simulink model "simulator_PID"  (R2024b)
settings: Solver=FixedStepAuto  StartTime=0.0  StopTime=100  FixedStep=0.01  RelTol=1e-3
values from neighbouring files (symbols this model uses):
  g = system_params.g    [system_model_quarternions.m]    (also in system_model_quat_omega.m)
  m = size(B,2)    [discretize_system.m]    (also in linearize_system.m = length(u0); linearize_system_euler.m = length(u0); model_init.m = system_params.m; system_model_quarternions.m = system_params.m)
  q0 = [0; 0; 0]    [model_init.m]    (also in test_model.m = x_test(1:3))
  qdot0 = [0;0;0]    [model_init.m]
  W_inv = inv(system_params.W)    [model_init.m]
undefined symbols (not defined in the file or in its folder): ALR, AUR, FD, LD, Lh, PLR, PUR, RD, W
libraries: slpidlib x5
settings Model: Creator=Sigbjørn  LastModifiedBy=Sigbjørn

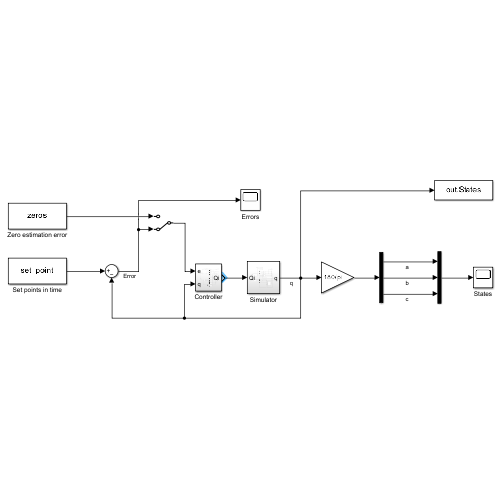
[thumbnail: Simulink's stored preview of the top-level diagram]
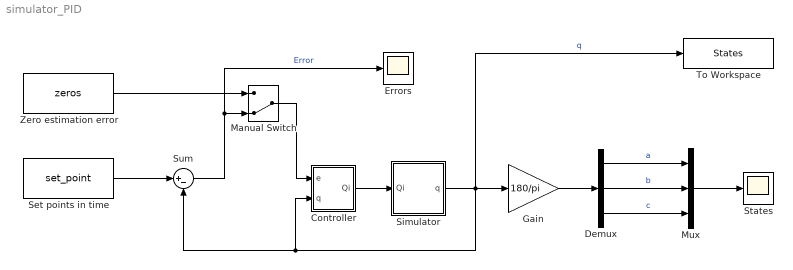
== system simulator_PID ==
  Controller : Subsystem
  Demux : Demux  Outputs=3
  Errors : Scope
  Gain : Gain  Gain=180/pi
  Manual Switch : ManualSwitch  CurrentSetting=0
  Mux : Mux  Inputs=3
  Set points in time : FromWorkspace  VariableName=set_point
  Simulator : Subsystem
  States : Scope
  Sum : Sum  Inputs=|+-
  To Workspace : ToWorkspace  VariableName=States  SaveFormat=Timeseries  SampleTime=-1
  Zero estimation error : FromWorkspace  VariableName=zeros
  wires:
  Set points in time/1 -> Sum/1
  Controller/1(Qi) -> Simulator/1(Qi)
  Sum/1 -> Manual Switch/2, Errors/1  "Error"
  Simulator/1(q) -> To Workspace/1, Gain/1, Controller/2(q), Sum/2  "q"
  Demux/1 -> Mux/1  "a"
  Demux/2 -> Mux/2  "b"
  Demux/3 -> Mux/3  "c"
  Zero estimation error/1 -> Manual Switch/1
  Manual Switch/1 -> Controller/1(e)
  Gain/1 -> Demux/1
  Mux/1 -> States/1

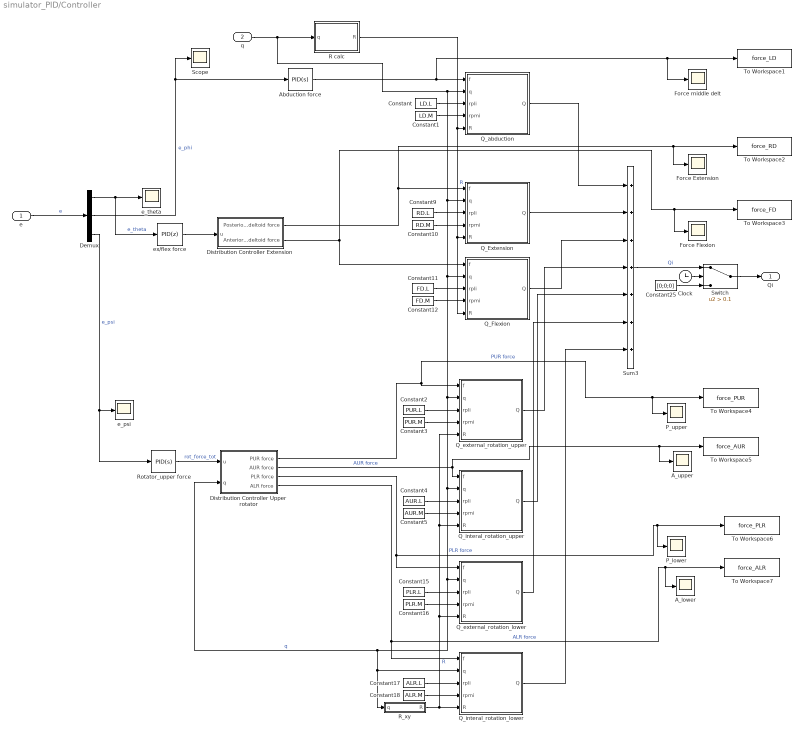
== system simulator_PID/Controller ==
  e : Inport
  q : Inport  Port=2
  A_lower : Scope
  A_upper : Scope
  Abduction force : slpidlib/PID Controller  Controller=PID  Form=Parallel  TimeDomain=Continuous-time  UseExternalTs=off  SampleTime=-1  IntegratorMethod=Forward Euler  FilterMethod=Forward Euler  ControllerParametersSource=internal  P=1  I=25  UseKiTs=off  D=5  UseExternalDerivativeSource=off  N=100  UseFilter=on  TunerSelectOption=Transfer Function Based (PID Tuner App)  InitialConditionSource=internal  InitialConditionForIntegrator=0  InitialConditionForFilter=0  DifferentiatorICPrevScaledInput=0  ExternalReset=none  TrackingMode=off  Kt=1  LimitOutput=on  SatLimitsSource=internal  UpperSaturationLimit=inf  LowerSaturationLimit=0  LinearizeAsGain=on  AntiWindupMode=none  Kb=1  LimitIntegrator=on  UpperIntegratorSaturationLimit=10000  LowerIntegratorSaturationLimit=0  POutMin=[]  POutMax=[]  IOutMin=[]  IOutMax=[]  DOutMin=[]  DOutMax=[]  NOutMin=[]  NOutMax=[]  SumOutMin=[]  SumOutMax=[]  SaturationOutMin=[]  SaturationOutMax=[]  PParamMin=[]  PParamMax=[]  IParamMin=[]  IParamMax=[]  DParamMin=[]  DParamMax=[]  NParamMin=[]  NParamMax=[]  KbParamMin=[]  KbParamMax=[]  KtParamMin=[]  KtParamMax=[]  KbOutMin=[]  KbOutMax=[]  KtOutMin=[]  KtOutMax=[]  IntegratorOutMin=[]  IntegratorOutMax=[]  FilterOutMin=[]  FilterOutMax=[]  SumI1OutMin=[]  SumI1OutMax=[]  SumI2OutMin=[]  SumI2OutMax=[]  SumI3OutMin=[]  SumI3OutMax=[]  SumI4OutMin=[]  SumI4OutMax=[]  SumDOutMin=[]  SumDOutMax=[]  DifferentiatorOutMin=[]  DifferentiatorOutMax=[]  FilterDiffOutCoefMin=[]  FilterDiffOutCoefMax=[]  ReciprocalOutMin=[]  ReciprocalOutMax=[]  SumDenOutMin=[]  SumDenOutMax=[]  SumNumOutMin=[]  SumNumOutMax=[]  DivideOutMin=[]  DivideOutMax=[]  UdiffTsProdOutMin=[]  UdiffTsProdOutMax=[]  NTsProdOutMin=[]  NTsProdOutMax=[]  UintegralTsProdOutMin=[]  UintegralTsProdOutMax=[]  UngainTsProdOutMin=[]  UngainTsProdOutMax=[]  ClampingZeroOutDataTypeStr=Inherit: Inherit via back propagation  ClampingZeroOutMin=[]  ClampingZeroOutMax=[]  FilterDenConstantOutDataTypeStr=Inherit: Inherit via back propagation  FilterDenConstantOutMin=[]  FilterDenConstantOutMax=[]  PCopyOutDataTypeStr=Inherit: Inherit via back propagation  PCopyOutMin=[]  PCopyOutMax=[]  NCopyOutDataTypeStr=Inherit: Inherit via back propagation  NCopyOutMin=[]  NCopyOutMax=[]  IntegratorContinuousStateAttributes=''  IntegratorStateMustResolveToSignalObject=off  IntegratorRTWStateStorageClass=Auto  FilterContinuousStateAttributes=''  FilterStateMustResolveToSignalObject=off  FilterRTWStateStorageClass=Auto  ParallelPVariant=InternalParameters  IdealPVariant=Disabled  IVariant=InternalParameters  DVariant=InternalParameters  IntegratorVariant=Continuous  SatVariant=Enabled  AWVariant=Passthrough  PCopyVariant=Disabled  TRVariant=Disabled  FdbkBlocksVariant=Forward  IdealPFdbkVariant=Disabled  SatFdbkVariant=Disabled  DerivativeFilterVariant=ContFilter  NVariant=InternalParameters  NCopyVariant=Disabled  FilterICVariant=InternalICsFilter  IntegratorICVariant=InternalICs  ExternalResetVariant=Disabled  TRSumVariant=Passthrough  SumFdbkVariant=Disabled  SumVariant=Sum_PID  TsampFilterVariant=InternalTs  TsampNgainVariant=Passthrough  TsampIntegralVariant=Disabled_SignalSpec  ExternalSaturationOutDataTypeStr=Inherit: Same as second input  DerivativeSourceVariant=ErrorSignal  PreIntVariant=InternalPreInt
  Clock : Clock
  Constant : Constant  Value=LD.L
  Constant1 : Constant  Value=LD.M
  Constant10 : Constant  Value=RD.M
  Constant11 : Constant  Value=FD.L
  Constant12 : Constant  Value=FD.M
  Constant15 : Constant  Value=PLR.L
  Constant16 : Constant  Value=PLR.M
  Constant17 : Constant  Value=ALR.L
  Constant18 : Constant  Value=ALR.M
  Constant2 : Constant  Value=PUR.L
  Constant25 : Constant  Value=[0;0;0]
  Constant3 : Constant  Value=PUR.M
  Constant4 : Constant  Value=AUR.L
  Constant5 : Constant  Value=AUR.M
  Constant9 : Constant  Value=RD.L
  Demux : Demux  Outputs=3
  Distribution Controller Extension : Subsystem
  Distribution Controller Upper rotator : Subsystem
  Force Extension : Scope
  Force Flexion : Scope
  Force middle delt : Scope
  P_lower : Scope
  P_upper : Scope
  Q_Extension : MATLAB Function  TreatAsAtomicUnit=on
  Q_Flexion : MATLAB Function  TreatAsAtomicUnit=on
  Q_abduction : MATLAB Function  TreatAsAtomicUnit=on
  Q_external_rotation_lower : MATLAB Function  TreatAsAtomicUnit=on
  Q_external_rotation_upper : MATLAB Function  TreatAsAtomicUnit=on
  Q_interal_rotation_lower : MATLAB Function  TreatAsAtomicUnit=on
  Q_interal_rotation_upper : MATLAB Function  TreatAsAtomicUnit=on
  R calc : MATLAB Function  TreatAsAtomicUnit=on
  R_xy : MATLAB Function  TreatAsAtomicUnit=on
  Rotator_upper force : slpidlib/PID Controller  Controller=PID  Form=Parallel  TimeDomain=Continuous-time  UseExternalTs=off  SampleTime=-1  IntegratorMethod=Forward Euler  FilterMethod=Forward Euler  ControllerParametersSource=internal  P=100  I=200  UseKiTs=off  D=500  UseExternalDerivativeSource=off  N=100  UseFilter=on  TunerSelectOption=Transfer Function Based (PID Tuner App)  InitialConditionSource=internal  InitialConditionForIntegrator=0  InitialConditionForFilter=0  DifferentiatorICPrevScaledInput=0  ExternalReset=none  TrackingMode=off  Kt=1  LimitOutput=on  SatLimitsSource=internal  UpperSaturationLimit=inf  LowerSaturationLimit=-inf  LinearizeAsGain=on  AntiWindupMode=none  Kb=1  LimitIntegrator=on  UpperIntegratorSaturationLimit=inf  LowerIntegratorSaturationLimit=-inf  POutMin=[]  POutMax=[]  IOutMin=[]  IOutMax=[]  DOutMin=[]  DOutMax=[]  NOutMin=[]  NOutMax=[]  SumOutMin=[]  SumOutMax=[]  SaturationOutMin=[]  SaturationOutMax=[]  PParamMin=[]  PParamMax=[]  IParamMin=[]  IParamMax=[]  DParamMin=[]  DParamMax=[]  NParamMin=[]  NParamMax=[]  KbParamMin=[]  KbParamMax=[]  KtParamMin=[]  KtParamMax=[]  KbOutMin=[]  KbOutMax=[]  KtOutMin=[]  KtOutMax=[]  IntegratorOutMin=[]  IntegratorOutMax=[]  FilterOutMin=[]  FilterOutMax=[]  SumI1OutMin=[]  SumI1OutMax=[]  SumI2OutMin=[]  SumI2OutMax=[]  SumI3OutMin=[]  SumI3OutMax=[]  SumI4OutMin=[]  SumI4OutMax=[]  SumDOutMin=[]  SumDOutMax=[]  DifferentiatorOutMin=[]  DifferentiatorOutMax=[]  FilterDiffOutCoefMin=[]  FilterDiffOutCoefMax=[]  ReciprocalOutMin=[]  ReciprocalOutMax=[]  SumDenOutMin=[]  SumDenOutMax=[]  SumNumOutMin=[]  SumNumOutMax=[]  DivideOutMin=[]  DivideOutMax=[]  UdiffTsProdOutMin=[]  UdiffTsProdOutMax=[]  NTsProdOutMin=[]  NTsProdOutMax=[]  UintegralTsProdOutMin=[]  UintegralTsProdOutMax=[]  UngainTsProdOutMin=[]  UngainTsProdOutMax=[]  ClampingZeroOutDataTypeStr=Inherit: Inherit via back propagation  ClampingZeroOutMin=[]  ClampingZeroOutMax=[]  FilterDenConstantOutDataTypeStr=Inherit: Inherit via back propagation  FilterDenConstantOutMin=[]  FilterDenConstantOutMax=[]  PCopyOutDataTypeStr=Inherit: Inherit via back propagation  PCopyOutMin=[]  PCopyOutMax=[]  NCopyOutDataTypeStr=Inherit: Inherit via back propagation  NCopyOutMin=[]  NCopyOutMax=[]  IntegratorContinuousStateAttributes=''  IntegratorStateMustResolveToSignalObject=off  IntegratorRTWStateStorageClass=Auto  FilterContinuousStateAttributes=''  FilterStateMustResolveToSignalObject=off  FilterRTWStateStorageClass=Auto  ParallelPVariant=InternalParameters  IdealPVariant=Disabled  IVariant=InternalParameters  DVariant=InternalParameters  IntegratorVariant=Continuous  SatVariant=Enabled  AWVariant=Passthrough  PCopyVariant=Disabled  TRVariant=Disabled  FdbkBlocksVariant=Forward  IdealPFdbkVariant=Disabled  SatFdbkVariant=Disabled  DerivativeFilterVariant=ContFilter  NVariant=InternalParameters  NCopyVariant=Disabled  FilterICVariant=InternalICsFilter  IntegratorICVariant=InternalICs  ExternalResetVariant=Disabled  TRSumVariant=Passthrough  SumFdbkVariant=Disabled  SumVariant=Sum_PID  TsampFilterVariant=InternalTs  TsampNgainVariant=Passthrough  TsampIntegralVariant=Disabled_SignalSpec  ExternalSaturationOutDataTypeStr=Inherit: Same as second input  DerivativeSourceVariant=ErrorSignal  PreIntVariant=InternalPreInt
  Scope : Scope
  Sum3 : Sum  Inputs=+++++++  InputSameDT=on  SaturateOnIntegerOverflow=on  OutDataTypeStr=Inherit: Same as first input
  Switch : Switch  Criteria=u2 > Threshold  Threshold=0.1  SaturateOnIntegerOverflow=off  InputSameDT=off
  To Workspace1 : ToWorkspace  VariableName=force_LD  SaveFormat=Timeseries  SampleTime=-1
  To Workspace2 : ToWorkspace  VariableName=force_RD  SaveFormat=Timeseries  SampleTime=-1
  To Workspace3 : ToWorkspace  VariableName=force_FD  SaveFormat=Timeseries  SampleTime=-1
  To Workspace4 : ToWorkspace  VariableName=force_PUR  SaveFormat=Timeseries  SampleTime=-1
  To Workspace5 : ToWorkspace  VariableName=force_AUR  SaveFormat=Timeseries  SampleTime=-1
  To Workspace6 : ToWorkspace  VariableName=force_PLR  SaveFormat=Timeseries  SampleTime=-1
  To Workspace7 : ToWorkspace  VariableName=force_ALR  SaveFormat=Timeseries  SampleTime=-1
  e_psi : Scope
  e_theta : Scope
  ex/flex force : slpidlib/PID Controller  Controller=PID  Form=Parallel  TimeDomain=Discrete-time  UseExternalTs=off  SampleTime=-1  IntegratorMethod=Forward Euler  FilterMethod=Forward Euler  ControllerParametersSource=internal  P=1  I=25  UseKiTs=off  D=5  UseExternalDerivativeSource=off  N=100  UseFilter=on  TunerSelectOption=Transfer Function Based (PID Tuner App)  InitialConditionSource=internal  InitialConditionForIntegrator=0  InitialConditionForFilter=0  DifferentiatorICPrevScaledInput=0  ExternalReset=none  TrackingMode=off  Kt=1  LimitOutput=on  SatLimitsSource=internal  UpperSaturationLimit=inf  LowerSaturationLimit=-inf  LinearizeAsGain=on  AntiWindupMode=none  Kb=1  LimitIntegrator=on  UpperIntegratorSaturationLimit=inf  LowerIntegratorSaturationLimit=-inf  POutMin=[]  POutMax=[]  IOutMin=[]  IOutMax=[]  DOutMin=[]  DOutMax=[]  NOutMin=[]  NOutMax=[]  SumOutMin=[]  SumOutMax=[]  SaturationOutMin=[]  SaturationOutMax=[]  PParamMin=[]  PParamMax=[]  IParamMin=[]  IParamMax=[]  DParamMin=[]  DParamMax=[]  NParamMin=[]  NParamMax=[]  KbParamMin=[]  KbParamMax=[]  KtParamMin=[]  KtParamMax=[]  KbOutMin=[]  KbOutMax=[]  KtOutMin=[]  KtOutMax=[]  IntegratorOutMin=[]  IntegratorOutMax=[]  FilterOutMin=[]  FilterOutMax=[]  SumI1OutMin=[]  SumI1OutMax=[]  SumI2OutMin=[]  SumI2OutMax=[]  SumI3OutMin=[]  SumI3OutMax=[]  SumI4OutMin=[]  SumI4OutMax=[]  SumDOutMin=[]  SumDOutMax=[]  DifferentiatorOutMin=[]  DifferentiatorOutMax=[]  FilterDiffOutCoefMin=[]  FilterDiffOutCoefMax=[]  ReciprocalOutMin=[]  ReciprocalOutMax=[]  SumDenOutMin=[]  SumDenOutMax=[]  SumNumOutMin=[]  SumNumOutMax=[]  DivideOutMin=[]  DivideOutMax=[]  UdiffTsProdOutMin=[]  UdiffTsProdOutMax=[]  NTsProdOutMin=[]  NTsProdOutMax=[]  UintegralTsProdOutMin=[]  UintegralTsProdOutMax=[]  UngainTsProdOutMin=[]  UngainTsProdOutMax=[]  ClampingZeroOutDataTypeStr=Inherit: Inherit via back propagation  ClampingZeroOutMin=[]  ClampingZeroOutMax=[]  FilterDenConstantOutDataTypeStr=Inherit: Inherit via back propagation  FilterDenConstantOutMin=[]  FilterDenConstantOutMax=[]  PCopyOutDataTypeStr=Inherit: Inherit via back propagation  PCopyOutMin=[]  PCopyOutMax=[]  NCopyOutDataTypeStr=Inherit: Inherit via back propagation  NCopyOutMin=[]  NCopyOutMax=[]  IntegratorContinuousStateAttributes=''  IntegratorStateMustResolveToSignalObject=off  IntegratorRTWStateStorageClass=Auto  FilterContinuousStateAttributes=''  FilterStateMustResolveToSignalObject=off  FilterRTWStateStorageClass=Auto  ParallelPVariant=InternalParameters  IdealPVariant=Disabled  IVariant=InternalParameters  DVariant=InternalParameters  IntegratorVariant=Discrete  SatVariant=Enabled  AWVariant=Passthrough  PCopyVariant=Disabled  TRVariant=Disabled  FdbkBlocksVariant=Forward  IdealPFdbkVariant=Disabled  SatFdbkVariant=Disabled  DerivativeFilterVariant=ForwardEulerFilter  NVariant=InternalParameters  NCopyVariant=Disabled  FilterICVariant=InternalICsFilter  IntegratorICVariant=InternalICs  ExternalResetVariant=Disabled  TRSumVariant=Passthrough  SumFdbkVariant=Disabled  SumVariant=Sum_PID  TsampFilterVariant=InternalTs  TsampNgainVariant=Passthrough  TsampIntegralVariant=Disabled_SignalSpec  ExternalSaturationOutDataTypeStr=Inherit: Same as second input  DerivativeSourceVariant=ErrorSignal  PreIntVariant=InternalPreInt
  Qi : Outport
  wires:
  q/1 -> Q_abduction/2(q), Q_Extension/2(q), Q_Flexion/2(q), Q_interal_rotation_lower/2(q), R_xy/1(q), Distribution Controller Upper rotator/2(q), Q_external_rotation_lower/2(q), Q_interal_rotation_upper/2(q), Q_external_rotation_upper/2(q), R calc/1(q)  "q"
  R calc/1(R) -> Q_Extension/5(R), Q_Flexion/5(R), Q_abduction/5(R)  "R"
  Constant/1 -> Q_abduction/3(rpli)
  Constant1/1 -> Q_abduction/4(rpmi)
  Sum3/1 -> Switch/1  "Qi"
  Demux/1 -> ex/flex force/1, e_theta/1  "e_theta"
  Demux/2 -> Scope/1, Abduction force/1  "e_phi"
  Demux/3 -> Rotator_upper force/1, e_psi/1  "e_psi"
  Constant2/1 -> Q_external_rotation_upper/3(rpli)
  Constant3/1 -> Q_external_rotation_upper/4(rpmi)
  Constant4/1 -> Q_interal_rotation_upper/3(rpli)
  Constant5/1 -> Q_interal_rotation_upper/4(rpmi)
  Q_abduction/1(Q) -> Sum3/1
  Q_interal_rotation_upper/1(Q) -> Sum3/5
  Q_external_rotation_upper/1(Q) -> Sum3/4
  Rotator_upper force/1 -> Distribution Controller Upper rotator/1(u)  "rot_force_tot"
  ex/flex force/1 -> Distribution Controller Extension/1(u)
  Constant9/1 -> Q_Extension/3(rpli)
  Constant10/1 -> Q_Extension/4(rpmi)
  Constant11/1 -> Q_Flexion/3(rpli)
  Constant12/1 -> Q_Flexion/4(rpmi)
  Q_Flexion/1(Q) -> Sum3/3
  Q_Extension/1(Q) -> Sum3/2
  Abduction force/1 -> Force middle delt/1, To Workspace1/1, Q_abduction/1(f)
  Distribution Controller Extension/1(Posterior deltoid force) -> To Workspace2/1, Force Extension/1, Q_Extension/1(f)
  Distribution Controller Extension/2(Anterior deltoid force) -> Q_Flexion/1(f), To Workspace3/1, Force Flexion/1
  Q_external_rotation_lower/1(Q) -> Sum3/6
  Q_interal_rotation_lower/1(Q) -> Sum3/7
  Constant15/1 -> Q_external_rotation_lower/3(rpli)
  Constant16/1 -> Q_external_rotation_lower/4(rpmi)
  Constant17/1 -> Q_interal_rotation_lower/3(rpli)
  Constant18/1 -> Q_interal_rotation_lower/4(rpmi)
  e/1 -> Demux/1  "e"
  Clock/1 -> Switch/2
  Constant25/1 -> Switch/3
  Switch/1 -> Qi/1
  Distribution Controller Upper rotator/4(ALR force) -> To Workspace7/1, A_lower/1, Q_interal_rotation_lower/1(f)  "ALR force"
  Distribution Controller Upper rotator/3(PLR force) -> To Workspace6/1, P_lower/1, Q_external_rotation_lower/1(f)  "PLR force"
  Distribution Controller Upper rotator/2(AUR force) -> A_upper/1, To Workspace5/1, Q_interal_rotation_upper/1(f)  "AUR force"
  Distribution Controller Upper rotator/1(PUR force) -> To Workspace4/1, P_upper/1, Q_external_rotation_upper/1(f)  "PUR force"
  R_xy/1(R) -> Q_external_rotation_upper/5(R), Q_interal_rotation_upper/5(R), Q_external_rotation_lower/5(R), Q_interal_rotation_lower/5(R)  "R"

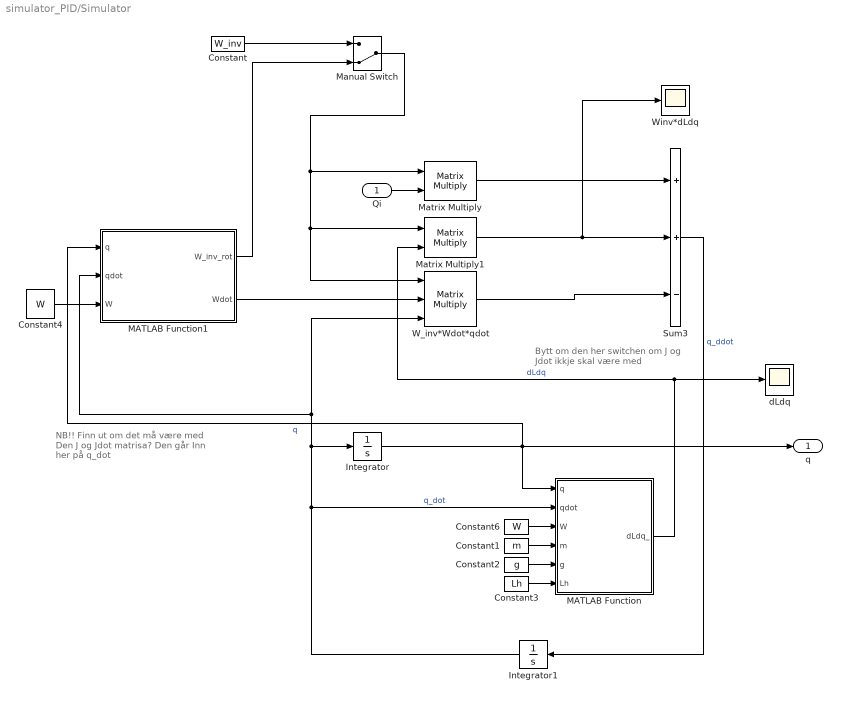
== system simulator_PID/Simulator ==
  note: Bytt om den her switchen
      | om J og Jdot ikkje skal være med
  note: NB!! Finn ut om det må være med
      | Den J og Jdot matrisa? Den går
      | Inn her på q_dot
  Qi : Inport
  Constant : Constant  Value=W_inv
  Constant1 : Constant  Value=m
  Constant2 : Constant  Value=g
  Constant3 : Constant  Value=Lh
  Constant4 : Constant  Value=W
  Constant6 : Constant  Value=W
  Integrator : Integrator  InitialCondition=q0
  Integrator1 : Integrator  InitialCondition=qdot0
  MATLAB Function : MATLAB Function  TreatAsAtomicUnit=on
  MATLAB Function1 : MATLAB Function  TreatAsAtomicUnit=on
  Manual Switch : ManualSwitch  CurrentSetting=0
  Matrix Multiply : Product  Multiplication=Matrix(*)
  Matrix Multiply1 : Product  Multiplication=Matrix(*)
  Sum3 : Sum  Inputs=++-  InputSameDT=on  SaturateOnIntegerOverflow=on  OutDataTypeStr=Inherit: Same as first input
  W_inv*Wdot*qdot : Product  Inputs=3  Multiplication=Matrix(*)
  Winv*dLdq : Scope
  dLdq : Scope
  q : Outport
  wires:
  Qi/1 -> Matrix Multiply/2
  Constant1/1 -> MATLAB Function/4(m)
  Constant2/1 -> MATLAB Function/5(g)
  Constant3/1 -> MATLAB Function/6(Lh)
  Integrator/1 -> MATLAB Function1/1(q), q/1, MATLAB Function/1(q)  "q"
  Integrator1/1 -> W_inv*Wdot*qdot/3, MATLAB Function1/2(qdot), Integrator/1, MATLAB Function/2(qdot)  "q_dot"
  MATLAB Function/1(dLdq_) -> dLdq/1, Matrix Multiply1/2  "dLdq"
  Sum3/1 -> Integrator1/1  "q_ddot"
  Matrix Multiply/1 -> Sum3/1
  Matrix Multiply1/1 -> Winv*dLdq/1, Sum3/2
  Constant/1 -> Manual Switch/1
  MATLAB Function1/2(Wdot) -> W_inv*Wdot*qdot/2
  MATLAB Function1/1(W_inv_rot) -> Manual Switch/2
  Manual Switch/1 -> W_inv*Wdot*qdot/1, Matrix Multiply1/1, Matrix Multiply/1
  Constant4/1 -> MATLAB Function1/3(W)
  W_inv*Wdot*qdot/1 -> Sum3/3
  Constant6/1 -> MATLAB Function/3(W)

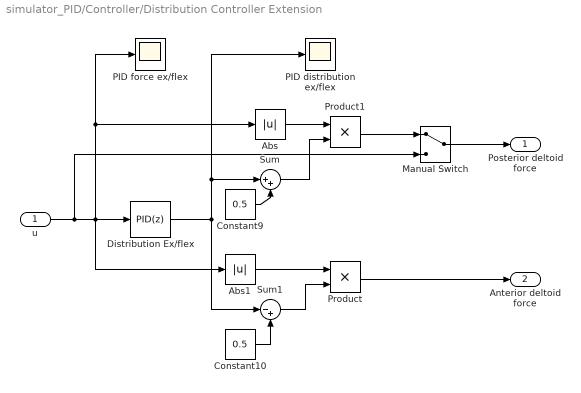
== system simulator_PID/Controller/Distribution Controller Extension ==
  u : Inport
  Abs : Abs  SaturateOnIntegerOverflow=off
  Abs1 : Abs  SaturateOnIntegerOverflow=off
  Constant10 : Constant  Value=0.5
  Constant9 : Constant  Value=0.5
  Distribution Ex/flex : slpidlib/PID Controller  Controller=PID  Form=Parallel  TimeDomain=Discrete-time  UseExternalTs=off  SampleTime=-1  IntegratorMethod=Forward Euler  FilterMethod=Forward Euler  ControllerParametersSource=internal  P=100  I=0  UseKiTs=off  D=0  UseExternalDerivativeSource=off  N=100  UseFilter=on  TunerSelectOption=Transfer Function Based (PID Tuner App)  InitialConditionSource=internal  InitialConditionForIntegrator=0  InitialConditionForFilter=0  DifferentiatorICPrevScaledInput=0  ExternalReset=none  TrackingMode=off  Kt=1  LimitOutput=on  SatLimitsSource=internal  UpperSaturationLimit=0.45  LowerSaturationLimit=-0.45  LinearizeAsGain=on  AntiWindupMode=none  Kb=1  LimitIntegrator=on  UpperIntegratorSaturationLimit=10  LowerIntegratorSaturationLimit=0  POutMin=[]  POutMax=[]  IOutMin=[]  IOutMax=[]  DOutMin=[]  DOutMax=[]  NOutMin=[]  NOutMax=[]  SumOutMin=[]  SumOutMax=[]  SaturationOutMin=[]  SaturationOutMax=[]  PParamMin=[]  PParamMax=[]  IParamMin=[]  IParamMax=[]  DParamMin=[]  DParamMax=[]  NParamMin=[]  NParamMax=[]  KbParamMin=[]  KbParamMax=[]  KtParamMin=[]  KtParamMax=[]  KbOutMin=[]  KbOutMax=[]  KtOutMin=[]  KtOutMax=[]  IntegratorOutMin=[]  IntegratorOutMax=[]  FilterOutMin=[]  FilterOutMax=[]  SumI1OutMin=[]  SumI1OutMax=[]  SumI2OutMin=[]  SumI2OutMax=[]  SumI3OutMin=[]  SumI3OutMax=[]  SumI4OutMin=[]  SumI4OutMax=[]  SumDOutMin=[]  SumDOutMax=[]  DifferentiatorOutMin=[]  DifferentiatorOutMax=[]  FilterDiffOutCoefMin=[]  FilterDiffOutCoefMax=[]  ReciprocalOutMin=[]  ReciprocalOutMax=[]  SumDenOutMin=[]  SumDenOutMax=[]  SumNumOutMin=[]  SumNumOutMax=[]  DivideOutMin=[]  DivideOutMax=[]  UdiffTsProdOutMin=[]  UdiffTsProdOutMax=[]  NTsProdOutMin=[]  NTsProdOutMax=[]  UintegralTsProdOutMin=[]  UintegralTsProdOutMax=[]  UngainTsProdOutMin=[]  UngainTsProdOutMax=[]  ClampingZeroOutDataTypeStr=Inherit: Inherit via back propagation  ClampingZeroOutMin=[]  ClampingZeroOutMax=[]  FilterDenConstantOutDataTypeStr=Inherit: Inherit via back propagation  FilterDenConstantOutMin=[]  FilterDenConstantOutMax=[]  PCopyOutDataTypeStr=Inherit: Inherit via back propagation  PCopyOutMin=[]  PCopyOutMax=[]  NCopyOutDataTypeStr=Inherit: Inherit via back propagation  NCopyOutMin=[]  NCopyOutMax=[]  IntegratorContinuousStateAttributes=''  IntegratorStateMustResolveToSignalObject=off  IntegratorRTWStateStorageClass=Auto  FilterContinuousStateAttributes=''  FilterStateMustResolveToSignalObject=off  FilterRTWStateStorageClass=Auto  ParallelPVariant=InternalParameters  IdealPVariant=Disabled  IVariant=InternalParameters  DVariant=InternalParameters  IntegratorVariant=Discrete  SatVariant=Enabled  AWVariant=Passthrough  PCopyVariant=Disabled  TRVariant=Disabled  FdbkBlocksVariant=Forward  IdealPFdbkVariant=Disabled  SatFdbkVariant=Disabled  DerivativeFilterVariant=ForwardEulerFilter  NVariant=InternalParameters  NCopyVariant=Disabled  FilterICVariant=InternalICsFilter  IntegratorICVariant=InternalICs  ExternalResetVariant=Disabled  TRSumVariant=Passthrough  SumFdbkVariant=Disabled  SumVariant=Sum_PID  TsampFilterVariant=InternalTs  TsampNgainVariant=Passthrough  TsampIntegralVariant=Disabled_SignalSpec  ExternalSaturationOutDataTypeStr=Inherit: Same as second input  DerivativeSourceVariant=ErrorSignal  PreIntVariant=InternalPreInt
  Manual Switch : ManualSwitch
  PID distribution ex/flex : Scope
  PID force ex/flex : Scope
  Product : Product
  Product1 : Product
  Sum : Sum  Inputs=|++
  Sum1 : Sum  Inputs=|-+
  Posterior deltoid force : Outport
  Anterior deltoid force : Outport  Port=2
  wires:
  Constant10/1 -> Sum1/2
  u/1 -> Manual Switch/2, Distribution Ex/flex/1, PID force ex/flex/1, Abs/1, Abs1/1
  Distribution Ex/flex/1 -> Sum1/1, PID distribution ex/flex/1, Sum/1
  Abs1/1 -> Product/1
  Sum/1 -> Product1/2
  Sum1/1 -> Product/2
  Abs/1 -> Product1/1
  Constant9/1 -> Sum/2
  Product1/1 -> Manual Switch/1
  Product/1 -> Anterior deltoid force/1
  Manual Switch/1 -> Posterior deltoid force/1

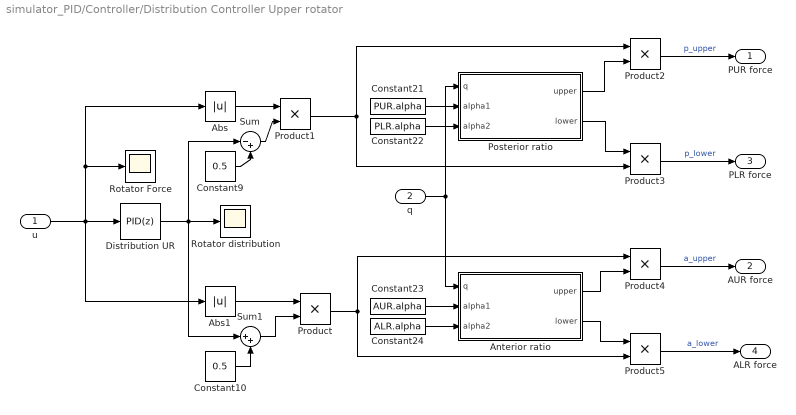
== system simulator_PID/Controller/Distribution Controller Upper rotator ==
  u : Inport
  q : Inport  Port=2
  Abs : Abs  SaturateOnIntegerOverflow=off
  Abs1 : Abs  SaturateOnIntegerOverflow=off
  Anterior ratio : MATLAB Function  TreatAsAtomicUnit=on
  Constant10 : Constant  Value=0.5
  Constant21 : Constant  Value=PUR.alpha
  Constant22 : Constant  Value=PLR.alpha
  Constant23 : Constant  Value=AUR.alpha
  Constant24 : Constant  Value=ALR.alpha
  Constant9 : Constant  Value=0.5
  Distribution UR : slpidlib/PID Controller  Controller=PID  Form=Parallel  TimeDomain=Discrete-time  UseExternalTs=off  SampleTime=-1  IntegratorMethod=Forward Euler  FilterMethod=Forward Euler  ControllerParametersSource=internal  P=100  I=0  UseKiTs=off  D=0  UseExternalDerivativeSource=off  N=100  UseFilter=on  TunerSelectOption=Transfer Function Based (PID Tuner App)  InitialConditionSource=internal  InitialConditionForIntegrator=0  InitialConditionForFilter=0  DifferentiatorICPrevScaledInput=0  ExternalReset=none  TrackingMode=off  Kt=1  LimitOutput=on  SatLimitsSource=internal  UpperSaturationLimit=0.45  LowerSaturationLimit=-0.45  LinearizeAsGain=on  AntiWindupMode=none  Kb=1  LimitIntegrator=on  UpperIntegratorSaturationLimit=10  LowerIntegratorSaturationLimit=0  POutMin=[]  POutMax=[]  IOutMin=[]  IOutMax=[]  DOutMin=[]  DOutMax=[]  NOutMin=[]  NOutMax=[]  SumOutMin=[]  SumOutMax=[]  SaturationOutMin=[]  SaturationOutMax=[]  PParamMin=[]  PParamMax=[]  IParamMin=[]  IParamMax=[]  DParamMin=[]  DParamMax=[]  NParamMin=[]  NParamMax=[]  KbParamMin=[]  KbParamMax=[]  KtParamMin=[]  KtParamMax=[]  KbOutMin=[]  KbOutMax=[]  KtOutMin=[]  KtOutMax=[]  IntegratorOutMin=[]  IntegratorOutMax=[]  FilterOutMin=[]  FilterOutMax=[]  SumI1OutMin=[]  SumI1OutMax=[]  SumI2OutMin=[]  SumI2OutMax=[]  SumI3OutMin=[]  SumI3OutMax=[]  SumI4OutMin=[]  SumI4OutMax=[]  SumDOutMin=[]  SumDOutMax=[]  DifferentiatorOutMin=[]  DifferentiatorOutMax=[]  FilterDiffOutCoefMin=[]  FilterDiffOutCoefMax=[]  ReciprocalOutMin=[]  ReciprocalOutMax=[]  SumDenOutMin=[]  SumDenOutMax=[]  SumNumOutMin=[]  SumNumOutMax=[]  DivideOutMin=[]  DivideOutMax=[]  UdiffTsProdOutMin=[]  UdiffTsProdOutMax=[]  NTsProdOutMin=[]  NTsProdOutMax=[]  UintegralTsProdOutMin=[]  UintegralTsProdOutMax=[]  UngainTsProdOutMin=[]  UngainTsProdOutMax=[]  ClampingZeroOutDataTypeStr=Inherit: Inherit via back propagation  ClampingZeroOutMin=[]  ClampingZeroOutMax=[]  FilterDenConstantOutDataTypeStr=Inherit: Inherit via back propagation  FilterDenConstantOutMin=[]  FilterDenConstantOutMax=[]  PCopyOutDataTypeStr=Inherit: Inherit via back propagation  PCopyOutMin=[]  PCopyOutMax=[]  NCopyOutDataTypeStr=Inherit: Inherit via back propagation  NCopyOutMin=[]  NCopyOutMax=[]  IntegratorContinuousStateAttributes=''  IntegratorStateMustResolveToSignalObject=off  IntegratorRTWStateStorageClass=Auto  FilterContinuousStateAttributes=''  FilterStateMustResolveToSignalObject=off  FilterRTWStateStorageClass=Auto  ParallelPVariant=InternalParameters  IdealPVariant=Disabled  IVariant=InternalParameters  DVariant=InternalParameters  IntegratorVariant=Discrete  SatVariant=Enabled  AWVariant=Passthrough  PCopyVariant=Disabled  TRVariant=Disabled  FdbkBlocksVariant=Forward  IdealPFdbkVariant=Disabled  SatFdbkVariant=Disabled  DerivativeFilterVariant=ForwardEulerFilter  NVariant=InternalParameters  NCopyVariant=Disabled  FilterICVariant=InternalICsFilter  IntegratorICVariant=InternalICs  ExternalResetVariant=Disabled  TRSumVariant=Passthrough  SumFdbkVariant=Disabled  SumVariant=Sum_PID  TsampFilterVariant=InternalTs  TsampNgainVariant=Passthrough  TsampIntegralVariant=Disabled_SignalSpec  ExternalSaturationOutDataTypeStr=Inherit: Same as second input  DerivativeSourceVariant=ErrorSignal  PreIntVariant=InternalPreInt
  Posterior ratio : MATLAB Function  TreatAsAtomicUnit=on
  Product{,1..5} (6 alike) : Product
  Rotator Force : Scope
  Rotator distribution : Scope
  Sum : Sum  Inputs=|-+
  Sum1 : Sum  Inputs=|++
  PUR force : Outport
  AUR force : Outport  Port=2
  PLR force : Outport  Port=3
  ALR force : Outport  Port=4
  wires:
  Constant10/1 -> Sum1/2
  u/1 -> Abs1/1, Distribution UR/1, Rotator Force/1, Abs/1
  Distribution UR/1 -> Rotator distribution/1, Sum1/1, Sum/1
  Abs1/1 -> Product/1
  Sum/1 -> Product1/2
  Sum1/1 -> Product/2
  Abs/1 -> Product1/1
  Constant9/1 -> Sum/2
  Posterior ratio/1(upper) -> Product2/2
  Constant24/1 -> Anterior ratio/3(alpha2)
  Constant23/1 -> Anterior ratio/2(alpha1)
  Anterior ratio/2(lower) -> Product5/1
  Product5/1 -> ALR force/1  "a_lower"
  q/1 -> Posterior ratio/1(q), Anterior ratio/1(q)
  Constant21/1 -> Posterior ratio/2(alpha1)
  Constant22/1 -> Posterior ratio/3(alpha2)
  Anterior ratio/1(upper) -> Product4/2
  Product/1 -> Product4/1, Product5/2
  Product2/1 -> PUR force/1  "p_upper"
  Posterior ratio/2(lower) -> Product3/1
  Product4/1 -> AUR force/1  "a_upper"
  Product1/1 -> Product3/2, Product2/1
  Product3/1 -> PLR force/1  "p_lower"

== matlab function simulator_PID/Controller/Q_external_rotation_lower ==
  data: f input; Q output; q input; rpli input; rpmi input; R input
function Q = fcn(f, q, rpli, rpmi, R)

Q = Qi(f, q, rpli, rpmi, R);

== matlab function simulator_PID/Controller/Q_interal_rotation_lower ==
  data: f input; Q output; q input; rpli input; rpmi input; R input
function Q = fcn(f, q, rpli, rpmi, R)

Q = Qi(f, q, rpli, rpmi, R);

== matlab function simulator_PID/Controller/Distribution Controller Upper rotator/Anterior ratio ==
  data: q input; upper output; alpha1 input; alpha2 input; lower output
function [upper, lower] = ul_rat(q, alpha1, alpha2)

[upper, lower] = ul_ratio(q, alpha1, alpha2);

== matlab function simulator_PID/Simulator/MATLAB Function1 ==
  data: q input; qdot input; W input; W_inv_rot output; Wdot output
function [W_inv_rot, Wdot] = W_Wdot_call(q, qdot, W)

[W_inv_rot, Wdot] = W_Wdot(q, qdot, W);

== matlab function simulator_PID/Controller/Distribution Controller Upper rotator/Posterior ratio ==
  data: q input; upper output; alpha1 input; alpha2 input; lower output
function [upper, lower] = ul_rat(q, alpha1, alpha2)

[upper, lower] = ul_ratio(q, alpha1, alpha2);

== matlab function simulator_PID/Simulator/MATLAB Function ==
  data: q input; qdot input; W input; dLdq_ output; m input; g input; Lh input
function dLdq_ = dLdq_call(q, qdot, W, m, g, Lh)
    dLdq_ = dLdq(q, qdot, W, m, g, Lh);
end

== matlab function simulator_PID/Controller/R calc ==
  data: q input; R output
function R = fcn(q)
R = Rot_mat(q);

== matlab function simulator_PID/Controller/Q_abduction ==
  data: f input; Q output; q input; rpli input; rpmi input; R input
function Q = fcn(f, q, rpli, rpmi, R)

Q = Qi(f, q, rpli, rpmi, R);

== matlab function simulator_PID/Controller/Q_external_rotation_upper ==
  data: f input; Q output; q input; rpli input; rpmi input; R input
function Q = fcn(f, q, rpli, rpmi, R)

Q = Qi(f, q, rpli, rpmi, R);

== matlab function simulator_PID/Controller/Q_interal_rotation_upper ==
  data: f input; Q output; q input; rpli input; rpmi input; R input
function Q = fcn(f, q, rpli, rpmi, R)

Q = Qi(f, q, rpli, rpmi, R);

== matlab function simulator_PID/Controller/Q_Extension ==
  data: f input; Q output; q input; rpli input; rpmi input; R input
function Q = fcn(f, q, rpli, rpmi, R)

Q = Qi(f, q, rpli, rpmi, R);

== matlab function simulator_PID/Controller/Q_Flexion ==
  data: f input; Q output; q input; rpli input; rpmi input; R input
function Q = fcn(f, q, rpli, rpmi, R)

Q = Qi(f, q, rpli, rpmi, R);

== matlab function simulator_PID/Controller/R_xy ==
  data: q input; R output
function R = fcn(q)
R = Rot_xy(q);
